simulink model "RRR_controller"  (R2020a)
settings: Solver=ode3  StartTime=0.0  StopTime=10  RelTol=1e-3
libraries: roblocks x11
settings Model: Creator=yrza  LastModifiedBy=Anuar

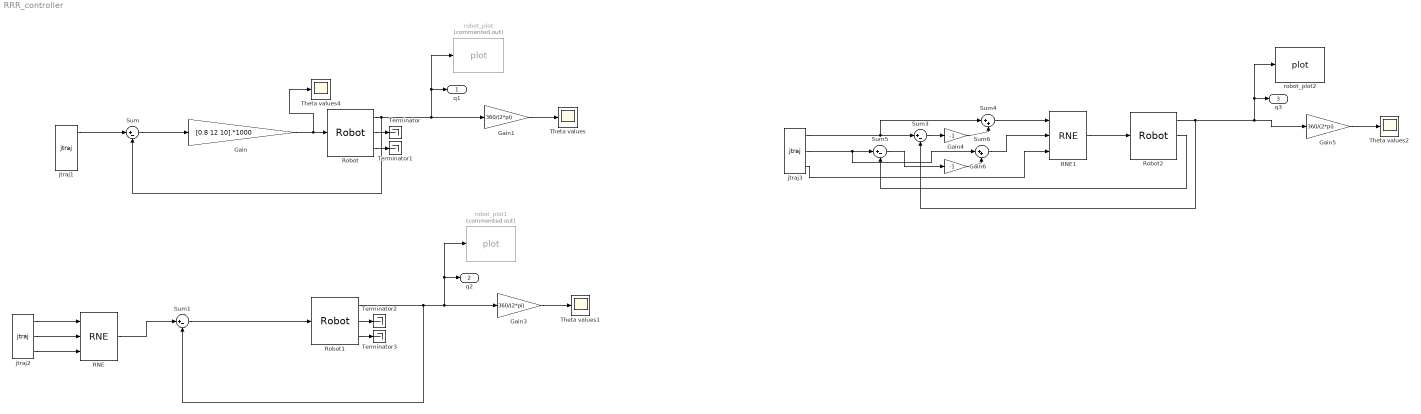
== system RRR_controller ==
  Gain : Gain  Gain=[0.8 12 10].*1000
  Gain1 : Gain  Gain=360/(2*pi)
  Gain3 : Gain  Gain=360/(2*pi)
  Gain4 : Gain  Gain=-1
  Gain5 : Gain  Gain=360/(2*pi)
  Gain6 : Gain  Gain=-1
  RNE : roblocks/Arm/RNE  robot=robot2  grav=[0 0 9.81]
  RNE1 : roblocks/Arm/RNE  robot=robot3  grav=[0 0 9.81]
  Robot : roblocks/Arm/Robot  robot=robot  q0=[0 0 0]
  Robot1 : roblocks/Arm/Robot  robot=robot2  q0=[0 0 0]
  Robot2 : roblocks/Arm/Robot  robot=robot3  q0=[0 0 0]
  Sum{,1,3,5} (4 alike) : Sum  Inputs=|+-
  Sum4 : Sum  Inputs=|++
  Sum6 : Sum  Inputs=|++
  Terminator{,1..3} (4 alike) : Terminator
  Theta values{,1..2,4} (4 alike) : Scope
  jtraj1 : roblocks/Toolbox/jtraj  q0=[0 0 0]  qf=[pi/2 -pi/4 -pi/4]  tmax=2.02  ts=0.02
  jtraj2 : roblocks/Toolbox/jtraj  q0=[0 0 0]  qf=[pi/2 -pi/4 -pi/4]  tmax=2.02  ts=0.02
  jtraj3 : roblocks/Toolbox/jtraj  q0=[0 0 0]  qf=[pi/2 -pi/4 -pi/4]  tmax=2.02  ts=0.02
  robot_plot : roblocks/Arm/plot  Commented=on  robot=robot  fps=5  holdplot=on
  robot_plot1 : roblocks/Arm/plot  Commented=on  robot=robot2  fps=5  holdplot=on
  robot_plot2 : roblocks/Arm/plot  robot=robot3  fps=5  holdplot=on
  q1 : Outport
  q2 : Outport  Port=2
  q3 : Outport  Port=3
  wires:
  Robot/1 -> robot_plot/1, q1/1, Gain1/1, Sum/2
  Gain/1 -> Theta values4/1, Robot/1
  Gain1/1 -> Theta values/1
  Sum/1 -> Gain/1
  Robot/2 -> Terminator/1
  Robot/3 -> Terminator1/1
  Sum1/1 -> Robot1/1
  Gain3/1 -> Theta values1/1
  Robot1/1 -> robot_plot1/1, q2/1, Gain3/1, Sum1/2
  jtraj2/1 -> RNE/1
  jtraj2/3 -> RNE/3
  jtraj2/2 -> RNE/2
  RNE/1 -> Sum1/1
  RNE1/1 -> Robot2/1
  Gain5/1 -> Theta values2/1
  Robot2/1 -> Sum3/2, robot_plot2/1, q3/1, Gain5/1
  jtraj3/1 -> Sum4/1, Sum3/1
  jtraj1/1 -> Sum/1
  Robot1/2 -> Terminator2/1
  Robot1/3 -> Terminator3/1
  jtraj3/3 -> RNE1/3
  Sum4/1 -> RNE1/1
  Sum3/1 -> Gain4/1
  Gain4/1 -> Sum4/2
  Robot2/2 -> Sum5/2
  jtraj3/2 -> Sum6/1, Sum5/1
  Gain6/1 -> Sum6/2
  Sum5/1 -> Gain6/1
  Sum6/1 -> RNE1/2
